simulink model "ACDCMG_woPV"  (R2020b)
settings: Solver=FixedStepAuto  StartTime=0.0  StopTime=0.2  FixedStep=Ts  MaxStep=1e-2  RelTol=1e-3
InitFcn:
  | Set_parameters_R2018
undefined symbols (not defined in the file): D1, D_invs, Delta, dis11, dis14, dis2, dis3, dis4, dis5, dis6, dis8, DiscIntNeverNeededParam, ee_sli_rtmsupport, fn, Fnom, gcbh, H_invs, Ion, Lithium, max_min, P_Load_3, P_nom_inv, Pnom_T1, Pnom_T2, Pnom_T3, Ql_Load_3, R_Load_9, R_Load_DC, Rl, Rls, S, sigbuilder_block, Ts, Ts_Control, Ts_Power, V1_LL_T3, VnInv, Vnom_DC, Vnom_Diesel, Vnom_prim, Vnom_sec, Vnom_ter_AC_DC, Xl, Xls
libraries: powerlib x238, powerlib_meascontrol x103, powerlib_extras x55, simulink x21, pid_lib x4, eeGeneralControl x2, re_lib x1, electricdrivelib x1, eeSinusoidalMeasurementV2 x1, eePowerMeasurement x1
(part 5 of 9)

== system ACDCMG_woPV/Grid Bi-directional Converter 1.2 300 (DC) // 150 V (AC) P_nom 3kW/Control of Inverter ==
  note: VL-L rms_2
  note: Primary control
  note: Control of Inverter
  Bus Selector : BusSelector  Commented=on  OutputSignals=signal1,signal2,signal3,signal4
  Demux3 : Demux  Outputs=3
  Demux4 : Demux  Outputs=3
  Discrete PWM Generator1 : Subsystem  Commented=on  AncestorBlock=|  DialogController=POWERSYS.PowerSysDialog  mask(Discrete PWM Generator){GeneratorMode=3-arm  bridge (6 pulses), Fc=4000, Ts=Ts_Power, Internal=off, mIndex=0.99, Freq=60, Phase=0}
      | powerlib_extras/Discrete 
      | Control Blocks/Discrete
      | PWM Generator
      mask prompts: GeneratorMode "Generator Mode"; Fc "Carrier frequency (Hz):"; Ts "Sample time:"; Internal "Internal generation of modulating signal(s)"; mIndex "Modulation index  (0<m<1) :"; Freq "Frequency of output voltage (Hz)"; Phase "Phase of output voltage (degrees)"
      mask help:
      | This discrete block generates pulses for carrier-based PWM (Pulse Width Modulation), self-commutated IGBTs,GTOs or FETs bridges.
      |
      | Depending on the number of bridge arms selected in the "Generator Mode" parameter, the block can be used either for single-phase or three-phase PWM control.
      mask init: same as ACDCMG_woPV/Grid Bi-directional Converter 1.1 300 (DC) // 150 V (AC) P_nom 3kW/Control of Inverter/Discrete PWM Generator1
      mask Help:
      | The output pulses are a vector (with values=0 or 1). Depending on the selected "Generator Mode", the output vector contains:
      | For a 1-arm  bridge: Two pulses. Pulse 1 is for the upper switch and pulse 2 is for the lower switch.
      | For a 2-arm  bridge: Four pulses. Pulses 1 and 3 are respectively for the upper switches of the first and second arm. Pulses 2 and 4 are for the lower switches.
      | For a 3-arm  bridge: Six pulses. Pulses 1,3 and 5 are respectively for the upper switches of the first,second and third arm. Pulses 2,4 and 6 are for the lower switches.
      | For double 3-arm bridges: Twelve pulses.The first six pulses (pulses 1 to 6) must be sent to the first 3-arm bridge and the last six (pulses 7 to 12) to the second 3-arm bridge.
      | 
      | By selecting "Internal generation" you can can control the modulation index m, frequency and phase of the output voltage  from the internal parameters (m, Freq and Phase). Otherwise, external signals are used for pulse generation. The width of the input vector must be 1 for single phase bridges ( 1-arm or 2-arm)  and 3 for 3-phase bridges  (single or double bridge).
      mask TypeOptions GeneratorMode: 1-arm  bridge (2 pulses) | 2-arm  bridge (4 pulses) | 3-arm  bridge (6 pulses) | Double 3-arm  bridges (12 pulses)
      mask Callback Internal: powericon('psbcallbacks',gcb,'Discrete PWM Generator',[]);
  Goto : Goto  Commented=on  GotoTag=PWM
  MI Controller : Subsystem  Commented=on
  Mux2 : Mux  Inputs=2
  PQ_B1 : Scope
  "P_Q(kW, kvar)1" : Display
      settings: Format=bank  Decimation=2000
  Positive-Sequence Active & Reactive Power1 : Subsystem  AncestorBlock=|  DialogController=POWERSYS.PowerSysDialog  mask(Discrete 3-phase Positive-Sequence Active & Reactive Power){Freq=60, Par_Vinit=[0 0], Par_Iinit=[0 0], Ts=5e-6}
      | powerlib_extras/Discrete
      | Measurements/Discrete 3-phase 
      | Positive-Sequence 
      | Active & Reactive Power
      mask prompts: Freq "Fundamental frequency (Hz):"; Par_Vinit "Voltage initial input: [ Mag  Phase(degrees) ]"; Par_Iinit "Current initial input: [ Mag  Phase(degrees) ]"; Ts "Sample time:"
      mask help:
      | Measure the three-phase active power P and reactive power Q associated with a periodic set of three-phase voltages and currents which may contain harmonics. P and Q are calculated by evaluating the fundamental values (positive-sequence) of the input voltages and currents with a running window over one cycle of the fundamental frequency.
      |
      | Current flowing into an RL circuit will produce  positive active and reactive powers.
      |
      | Vabc input: Three-phase instantaneous voltage (V)
      | Iabc input: Three-phase instantaneous current (A)
      |
      | Output 1: Vector [Mag_V(V) Mag_I(A)] of the fundamental values of the voltage & current (peak values of the positive-sequence)
      | Output 2: 3-phase PQ measurement vector [P(W) Q (var)] evaluated at the fundamental frequency.
      |
      | For the first cycle of simulation, the outputs are held constant using the values specified by the parameters "Initial input".
      mask init:
      | power_initmask();
      mask Help: This block is part of a subset of blocks in the Extras library that does not have documentation associated with it, other than the block mask description.
      mask Display: disp('')
  RMS_VI2 : Scope
  RMS_V_I1 : Display
      settings: Format=bank  Decimation=2000
  Scope1 : Scope  NumInputPorts=2
  Scope2 : Scope
  Scope6 : Scope  NumInputPorts=2
  Terminator{1..6} (6 alike) : Terminator
  Unit Delay4 : UnitDelay  Commented=on  SampleTime=Ts_Power  HasFrameUpgradeWarning=on
  V/F : Subsystem
  VL-L_2 : Scope  Commented=on  NumInputPorts=2
  Vph_rms_2 : Scope  Commented=on
  m2 : Scope  Commented=on
  m_2 : Scope  Commented=on
  Pulses : Outport  VectorParamsAs1DForOutWhenUnconnected=off
  wires:
  MI Controller/2(m) -> m_2/1
  Discrete PWM Generator1/1(Pulses) -> Unit Delay4/1
  MI Controller/1(Vabc_inv) -> Discrete PWM Generator1/1(Uref)
  Bus Selector/1 -> m2/1, MI Controller/1(Vabc)  "<signal1>"
  Bus Selector/2 -> VL-L_2/1  "<signal2>"
  Bus Selector/3 -> VL-L_2/2  "<signal3>"
  Bus Selector/4 -> Vph_rms_2/1  "<signal4>"
  [Udc] -> V/F/4(Udc)
  Demux3/2 -> Terminator1/1
  Demux4/3 -> Terminator6/1
  [i] -> V/F/3(i)
  Demux4/2 -> Terminator5/1
  Demux4/1 -> Mux2/2
  Demux3/3 -> Terminator4/1
  [io] -> Scope1/2, Positive-Sequence Active & Reactive Power1/2(Iabc)
  Mux2/1 -> Scope2/1
  Demux3/1 -> Mux2/1
  Positive-Sequence Active & Reactive Power1/2(P_Q(kW)) -> PQ_B1/1, "P_Q(kW, kvar)1"/1
  Positive-Sequence Active & Reactive Power1/4(PF) -> Terminator3/1
  Positive-Sequence Active & Reactive Power1/3(Phase_V_I) -> Terminator2/1
  Positive-Sequence Active & Reactive Power1/1(RMS_V_I) -> RMS_V_I1/1, RMS_VI2/1
  [e] -> Scope1/1, Positive-Sequence Active & Reactive Power1/1(Vabc)
  [e] -> Scope6/1, Demux3/1, V/F/1(e)
  [io] -> Scope6/2, Demux4/1, V/F/2(io)
  V/F/1(Pulses) -> Pulses/1

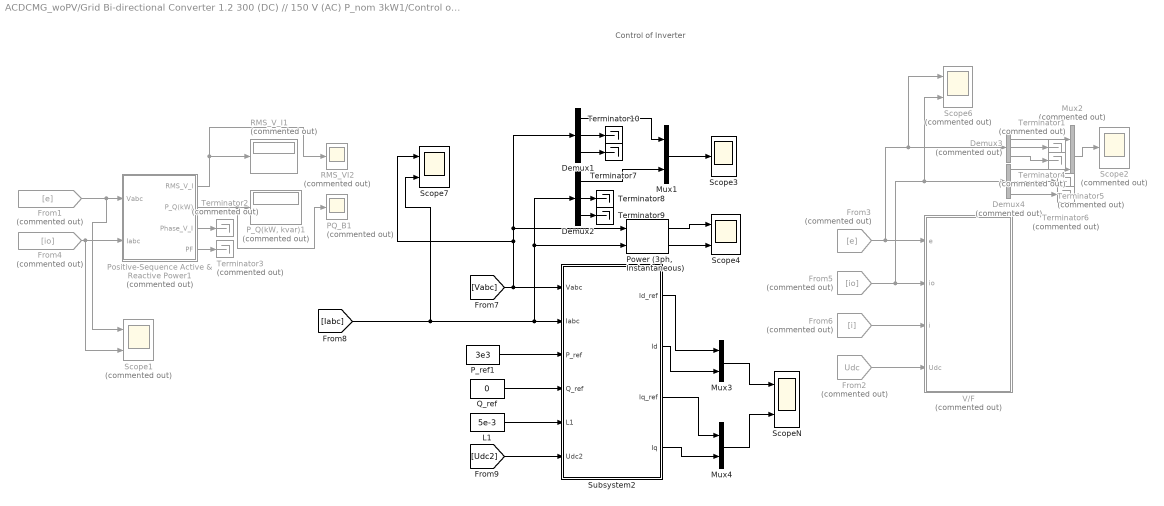
== system ACDCMG_woPV/Grid Bi-directional Converter 1.2 300 (DC) // 150 V (AC) P_nom 3kW1/Control of Inverter ==
  note: Control of Inverter
  Demux1 : Demux  Outputs=3
  Demux2 : Demux  Outputs=3
  Demux3 : Demux  Commented=on  Outputs=3
  Demux4 : Demux  Commented=on  Outputs=3
  From1 : From  Commented=on  GotoTag=e  TagVisibility=global
      settings: CloseFcn=tagdialog Close
  From2 : From  Commented=on  GotoTag=Udc  TagVisibility=global
  From3 : From  Commented=on  GotoTag=e  TagVisibility=global
  From4 : From  Commented=on  GotoTag=io  TagVisibility=global
      settings: CloseFcn=tagdialog Close
  From5 : From  Commented=on  GotoTag=io  TagVisibility=global
  From6 : From  Commented=on  GotoTag=i  TagVisibility=global
  L1 : Constant  Value=5e-3
  Mux1 : Mux  Inputs=2
  Mux2 : Mux  Commented=on  Inputs=2
  Mux3 : Mux  Inputs=2
  Mux4 : Mux  Inputs=2
  PQ_B1 : Scope  Commented=on
  "P_Q(kW, kvar)1" : Display  Commented=on
      settings: Format=bank  Decimation=2000
  P_ref1 : Constant  Value=3e3
  Positive-Sequence Active & Reactive Power1 : Subsystem  Commented=on  AncestorBlock=|  DialogController=POWERSYS.PowerSysDialog  mask(Discrete 3-phase Positive-Sequence Active & Reactive Power){Freq=60, Par_Vinit=[0 0], Par_Iinit=[0 0], Ts=5e-6}
      | powerlib_extras/Discrete
      | Measurements/Discrete 3-phase 
      | Positive-Sequence 
      | Active & Reactive Power
      mask prompts: Freq "Fundamental frequency (Hz):"; Par_Vinit "Voltage initial input: [ Mag  Phase(degrees) ]"; Par_Iinit "Current initial input: [ Mag  Phase(degrees) ]"; Ts "Sample time:"
      mask help:
      | Measure the three-phase active power P and reactive power Q associated with a periodic set of three-phase voltages and currents which may contain harmonics. P and Q are calculated by evaluating the fundamental values (positive-sequence) of the input voltages and currents with a running window over one cycle of the fundamental frequency.
      |
      | Current flowing into an RL circuit will produce  positive active and reactive powers.
      |
      | Vabc input: Three-phase instantaneous voltage (V)
      | Iabc input: Three-phase instantaneous current (A)
      |
      | Output 1: Vector [Mag_V(V) Mag_I(A)] of the fundamental values of the voltage & current (peak values of the positive-sequence)
      | Output 2: 3-phase PQ measurement vector [P(W) Q (var)] evaluated at the fundamental frequency.
      |
      | For the first cycle of simulation, the outputs are held constant using the values specified by the parameters "Initial input".
      mask init:
      | power_initmask();
      mask Help: This block is part of a subset of blocks in the Extras library that does not have documentation associated with it, other than the block mask description.
      mask Display: disp('')
  "Power (3ph, Instantaneous)" : powerlib_meascontrol/Measurements/Power (3ph, Instantaneous)
  Q_ref : Constant  Value=0
  RMS_VI2 : Scope  Commented=on
  RMS_V_I1 : Display  Commented=on
      settings: Format=bank  Decimation=2000
  Scope1 : Scope  Commented=on  NumInputPorts=2
  Scope2 : Scope  Commented=on
  Scope3 : Scope
  Scope4 : Scope  NumInputPorts=2
  Scope6 : Scope  Commented=on  NumInputPorts=2
  Scope7 : Scope  NumInputPorts=2
  ScopeN : Scope  NumInputPorts=2
  Subsystem2 : Subsystem  mask{Kp=21, Ki=101, Kd=0}
      mask prompts: Kp "Proportional gain (Kp):"; Ki "Integral gain (Ki):"; Kd "Derivative gain (Kd):"
  Terminator{1..6} (6 alike) : Terminator  Commented=on
  Terminator{7..10} (4 alike) : Terminator
  V/F : Subsystem  Commented=on
  wires:
  From2/1 -> V/F/4(Udc)
  Demux3/2 -> Terminator1/1
  Demux4/3 -> Terminator6/1
  From6/1 -> V/F/3(i)
  Demux4/2 -> Terminator5/1
  Demux4/1 -> Mux2/2
  Demux3/3 -> Terminator4/1
  From4/1 -> Scope1/2, Positive-Sequence Active & Reactive Power1/2(Iabc)
  Mux2/1 -> Scope2/1
  Demux3/1 -> Mux2/1
  Positive-Sequence Active & Reactive Power1/2(P_Q(kW)) -> PQ_B1/1, "P_Q(kW, kvar)1"/1
  Positive-Sequence Active & Reactive Power1/4(PF) -> Terminator3/1
  Positive-Sequence Active & Reactive Power1/3(Phase_V_I) -> Terminator2/1
  Positive-Sequence Active & Reactive Power1/1(RMS_V_I) -> RMS_V_I1/1, RMS_VI2/1
  From1/1 -> Scope1/1, Positive-Sequence Active & Reactive Power1/1(Vabc)
  From3/1 -> Scope6/1, Demux3/1, V/F/1(e)
  From5/1 -> Scope6/2, Demux4/1, V/F/2(io)
  Q_ref/1 -> Subsystem2/4(Q_ref)
  [Vabc] -> Subsystem2/1(Vabc), Scope7/1, Demux1/1, "Power (3ph, Instantaneous)"/1
  Demux2/3 -> Terminator9/1
  Demux1/2 -> Terminator10/1
  [Udc2] -> Subsystem2/6(Udc2)
  P_ref1/1 -> Subsystem2/3(P_ref)
  Demux2/2 -> Terminator8/1
  "Power (3ph, Instantaneous)"/2 -> Scope4/2
  "Power (3ph, Instantaneous)"/1 -> Scope4/1
  Subsystem2/3(Iq_ref) -> Mux4/1
  Subsystem2/2(Id) -> Mux3/2
  Demux2/1 -> Mux1/2
  Mux1/1 -> Scope3/1
  L1/1 -> Subsystem2/5(L1)
  Mux3/1 -> ScopeN/1
  Subsystem2/4(Iq) -> Mux4/2
  [Iabc] -> Scope7/2, Demux2/1, "Power (3ph, Instantaneous)"/2, Subsystem2/2(Iabc)
  Subsystem2/1(Id_ref) -> Mux3/1
  Mux4/1 -> ScopeN/2
  Demux1/3 -> Terminator7/1
  Demux1/1 -> Mux1/1

== system ACDCMG_woPV/Grid Bi-directional Converter 1.2 300 (DC) // 150 V (AC) P_nom 3kW1/Power Measurement (Three-Phase) ==
  V : Inport
  I : Inport  Port=2
  Continuous : Subsystem  VariantControl=Continuous
  Discrete : Subsystem  VariantControl=Discrete
  P : Outport  VectorParamsAs1DForOutWhenUnconnected=off
  Q : Outport  Port=2  VectorParamsAs1DForOutWhenUnconnected=off

== system ACDCMG_woPV/Grid Bi-directional Converter 1.2 300 (DC) // 150 V (AC) P_nom 3kW2/Control of Inverter ==
  note: VL-L rms_2
  note: Primary control
  note: Control of Inverter
  Bus Selector : BusSelector  Commented=on  OutputSignals=signal1,signal2,signal3,signal4
  Demux3 : Demux  Outputs=3
  Demux4 : Demux  Outputs=3
  Discrete PWM Generator1 : Subsystem  Commented=on  AncestorBlock=|  DialogController=POWERSYS.PowerSysDialog  mask(Discrete PWM Generator){GeneratorMode=3-arm  bridge (6 pulses), Fc=4000, Ts=Ts_Power, Internal=off, mIndex=0.99, Freq=60, Phase=0}
      | powerlib_extras/Discrete 
      | Control Blocks/Discrete
      | PWM Generator
      mask prompts: GeneratorMode "Generator Mode"; Fc "Carrier frequency (Hz):"; Ts "Sample time:"; Internal "Internal generation of modulating signal(s)"; mIndex "Modulation index  (0<m<1) :"; Freq "Frequency of output voltage (Hz)"; Phase "Phase of output voltage (degrees)"
      mask help:
      | This discrete block generates pulses for carrier-based PWM (Pulse Width Modulation), self-commutated IGBTs,GTOs or FETs bridges.
      |
      | Depending on the number of bridge arms selected in the "Generator Mode" parameter, the block can be used either for single-phase or three-phase PWM control.
      mask init: same as ACDCMG_woPV/Grid Bi-directional Converter 1.1 300 (DC) // 150 V (AC) P_nom 3kW/Control of Inverter/Discrete PWM Generator1
      mask Help:
      | The output pulses are a vector (with values=0 or 1). Depending on the selected "Generator Mode", the output vector contains:
      | For a 1-arm  bridge: Two pulses. Pulse 1 is for the upper switch and pulse 2 is for the lower switch.
      | For a 2-arm  bridge: Four pulses. Pulses 1 and 3 are respectively for the upper switches of the first and second arm. Pulses 2 and 4 are for the lower switches.
      | For a 3-arm  bridge: Six pulses. Pulses 1,3 and 5 are respectively for the upper switches of the first,second and third arm. Pulses 2,4 and 6 are for the lower switches.
      | For double 3-arm bridges: Twelve pulses.The first six pulses (pulses 1 to 6) must be sent to the first 3-arm bridge and the last six (pulses 7 to 12) to the second 3-arm bridge.
      | 
      | By selecting "Internal generation" you can can control the modulation index m, frequency and phase of the output voltage  from the internal parameters (m, Freq and Phase). Otherwise, external signals are used for pulse generation. The width of the input vector must be 1 for single phase bridges ( 1-arm or 2-arm)  and 3 for 3-phase bridges  (single or double bridge).
      mask TypeOptions GeneratorMode: 1-arm  bridge (2 pulses) | 2-arm  bridge (4 pulses) | 3-arm  bridge (6 pulses) | Double 3-arm  bridges (12 pulses)
      mask Callback Internal: powericon('psbcallbacks',gcb,'Discrete PWM Generator',[]);
  Goto : Goto  Commented=on  GotoTag=PWM
  MI Controller : Subsystem  Commented=on
  Mux2 : Mux  Inputs=2
  PQ_B1 : Scope
  "P_Q(kW, kvar)1" : Display
      settings: Format=bank  Decimation=2000
  Positive-Sequence Active & Reactive Power1 : Subsystem  AncestorBlock=|  DialogController=POWERSYS.PowerSysDialog  mask(Discrete 3-phase Positive-Sequence Active & Reactive Power){Freq=60, Par_Vinit=[0 0], Par_Iinit=[0 0], Ts=5e-6}
      | powerlib_extras/Discrete
      | Measurements/Discrete 3-phase 
      | Positive-Sequence 
      | Active & Reactive Power
      mask prompts: Freq "Fundamental frequency (Hz):"; Par_Vinit "Voltage initial input: [ Mag  Phase(degrees) ]"; Par_Iinit "Current initial input: [ Mag  Phase(degrees) ]"; Ts "Sample time:"
      mask help:
      | Measure the three-phase active power P and reactive power Q associated with a periodic set of three-phase voltages and currents which may contain harmonics. P and Q are calculated by evaluating the fundamental values (positive-sequence) of the input voltages and currents with a running window over one cycle of the fundamental frequency.
      |
      | Current flowing into an RL circuit will produce  positive active and reactive powers.
      |
      | Vabc input: Three-phase instantaneous voltage (V)
      | Iabc input: Three-phase instantaneous current (A)
      |
      | Output 1: Vector [Mag_V(V) Mag_I(A)] of the fundamental values of the voltage & current (peak values of the positive-sequence)
      | Output 2: 3-phase PQ measurement vector [P(W) Q (var)] evaluated at the fundamental frequency.
      |
      | For the first cycle of simulation, the outputs are held constant using the values specified by the parameters "Initial input".
      mask init:
      | power_initmask();
      mask Help: This block is part of a subset of blocks in the Extras library that does not have documentation associated with it, other than the block mask description.
      mask Display: disp('')
  RMS_VI2 : Scope
  RMS_V_I1 : Display
      settings: Format=bank  Decimation=2000
  Scope1 : Scope  NumInputPorts=2
  Scope2 : Scope
  Scope6 : Scope  NumInputPorts=2
  Terminator{1..6} (6 alike) : Terminator
  Unit Delay4 : UnitDelay  Commented=on  SampleTime=Ts_Power  HasFrameUpgradeWarning=on
  V/F : Subsystem
  VL-L_2 : Scope  Commented=on  NumInputPorts=2
  Vph_rms_2 : Scope  Commented=on
  m2 : Scope  Commented=on
  m_2 : Scope  Commented=on
  Pulses : Outport  VectorParamsAs1DForOutWhenUnconnected=off
  wires:
  MI Controller/2(m) -> m_2/1
  Discrete PWM Generator1/1(Pulses) -> Unit Delay4/1
  MI Controller/1(Vabc_inv) -> Discrete PWM Generator1/1(Uref)
  Bus Selector/1 -> m2/1, MI Controller/1(Vabc)  "<signal1>"
  Bus Selector/2 -> VL-L_2/1  "<signal2>"
  Bus Selector/3 -> VL-L_2/2  "<signal3>"
  Bus Selector/4 -> Vph_rms_2/1  "<signal4>"
  [Udc] -> V/F/4(Udc)
  Demux3/2 -> Terminator1/1
  Demux4/3 -> Terminator6/1
  [i] -> V/F/3(i)
  Demux4/2 -> Terminator5/1
  Demux4/1 -> Mux2/2
  Demux3/3 -> Terminator4/1
  [io] -> Scope1/2, Positive-Sequence Active & Reactive Power1/2(Iabc)
  Mux2/1 -> Scope2/1
  Demux3/1 -> Mux2/1
  Positive-Sequence Active & Reactive Power1/2(P_Q(kW)) -> PQ_B1/1, "P_Q(kW, kvar)1"/1
  Positive-Sequence Active & Reactive Power1/4(PF) -> Terminator3/1
  Positive-Sequence Active & Reactive Power1/3(Phase_V_I) -> Terminator2/1
  Positive-Sequence Active & Reactive Power1/1(RMS_V_I) -> RMS_V_I1/1, RMS_VI2/1
  [e] -> Scope1/1, Positive-Sequence Active & Reactive Power1/1(Vabc)
  [e] -> Scope6/1, Demux3/1, V/F/1(e)
  [io] -> Scope6/2, Demux4/1, V/F/2(io)
  V/F/1(Pulses) -> Pulses/1

== system ACDCMG_woPV/Grid Bi-directional Converter 1.2 300 (DC) // 150 V (AC) P_nom 3kW3/Control of Inverter ==
  note: Control of Inverter
  Demux3 : Demux  Outputs=3
  Demux4 : Demux  Outputs=3
  From1 : From  Commented=on  GotoTag=e  TagVisibility=global
      settings: CloseFcn=tagdialog Close
  From4 : From  Commented=on  GotoTag=io  TagVisibility=global
      settings: CloseFcn=tagdialog Close
  Mux2 : Mux  Inputs=2
  PQ_B1 : Scope  Commented=on
  "P_Q(kW, kvar)1" : Display  Commented=on
      settings: Format=bank  Decimation=2000
  Positive-Sequence Active & Reactive Power1 : Subsystem  Commented=on  AncestorBlock=|  DialogController=POWERSYS.PowerSysDialog  mask(Discrete 3-phase Positive-Sequence Active & Reactive Power){Freq=60, Par_Vinit=[0 0], Par_Iinit=[0 0], Ts=5e-6}
      | powerlib_extras/Discrete
      | Measurements/Discrete 3-phase 
      | Positive-Sequence 
      | Active & Reactive Power
      mask prompts: Freq "Fundamental frequency (Hz):"; Par_Vinit "Voltage initial input: [ Mag  Phase(degrees) ]"; Par_Iinit "Current initial input: [ Mag  Phase(degrees) ]"; Ts "Sample time:"
      mask help:
      | Measure the three-phase active power P and reactive power Q associated with a periodic set of three-phase voltages and currents which may contain harmonics. P and Q are calculated by evaluating the fundamental values (positive-sequence) of the input voltages and currents with a running window over one cycle of the fundamental frequency.
      |
      | Current flowing into an RL circuit will produce  positive active and reactive powers.
      |
      | Vabc input: Three-phase instantaneous voltage (V)
      | Iabc input: Three-phase instantaneous current (A)
      |
      | Output 1: Vector [Mag_V(V) Mag_I(A)] of the fundamental values of the voltage & current (peak values of the positive-sequence)
      | Output 2: 3-phase PQ measurement vector [P(W) Q (var)] evaluated at the fundamental frequency.
      |
      | For the first cycle of simulation, the outputs are held constant using the values specified by the parameters "Initial input".
      mask init:
      | power_initmask();
      mask Help: This block is part of a subset of blocks in the Extras library that does not have documentation associated with it, other than the block mask description.
      mask Display: disp('')
  RMS_VI2 : Scope  Commented=on
  RMS_V_I1 : Display  Commented=on
      settings: Format=bank  Decimation=2000
  Scope1 : Scope  Commented=on  NumInputPorts=2
  Scope2 : Scope
  Scope6 : Scope  NumInputPorts=2
  Terminator{1,4..6} (4 alike) : Terminator
  Terminator2 : Terminator  Commented=on
  Terminator3 : Terminator  Commented=on
  V/F : Subsystem
  wires:
  [Udc] -> V/F/4(Udc)
  Demux3/2 -> Terminator1/1
  Demux4/3 -> Terminator6/1
  [i] -> V/F/3(i)
  Demux4/2 -> Terminator5/1
  Demux4/1 -> Mux2/2
  Demux3/3 -> Terminator4/1
  From4/1 -> Scope1/2, Positive-Sequence Active & Reactive Power1/2(Iabc)
  Mux2/1 -> Scope2/1
  Demux3/1 -> Mux2/1
  Positive-Sequence Active & Reactive Power1/2(P_Q(kW)) -> PQ_B1/1, "P_Q(kW, kvar)1"/1
  Positive-Sequence Active & Reactive Power1/4(PF) -> Terminator3/1
  Positive-Sequence Active & Reactive Power1/3(Phase_V_I) -> Terminator2/1
  Positive-Sequence Active & Reactive Power1/1(RMS_V_I) -> RMS_V_I1/1, RMS_VI2/1
  From1/1 -> Scope1/1, Positive-Sequence Active & Reactive Power1/1(Vabc)
  [e] -> Scope6/1, Demux3/1, V/F/1(e)
  [io] -> Scope6/2, Demux4/1, V/F/2(io)

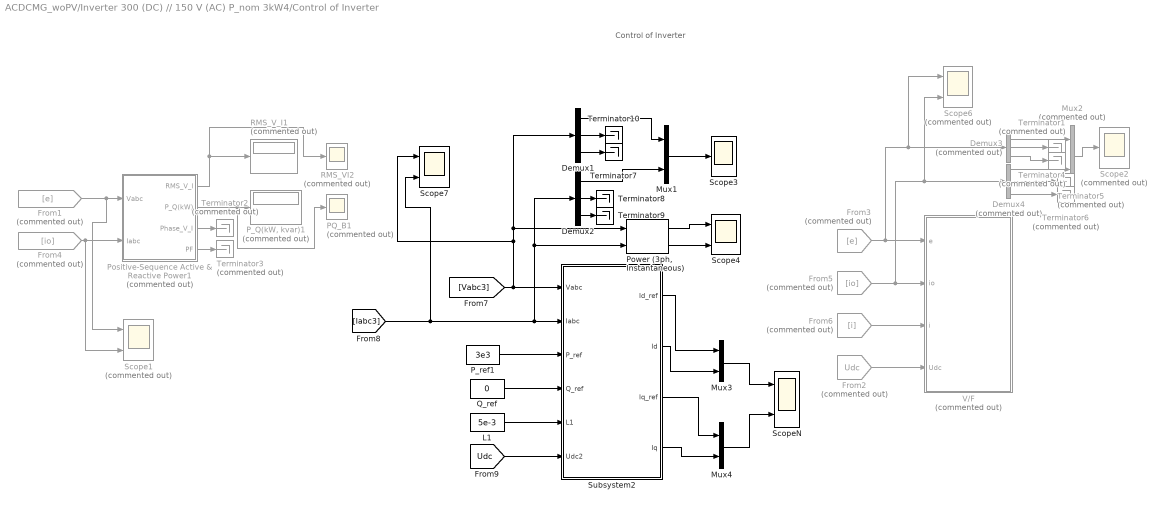
== system ACDCMG_woPV/Inverter 300 (DC) // 150 V (AC) P_nom 3kW4/Control of Inverter ==
  note: Control of Inverter
  Demux1 : Demux  Outputs=3
  Demux2 : Demux  Outputs=3
  Demux3 : Demux  Commented=on  Outputs=3
  Demux4 : Demux  Commented=on  Outputs=3
  From1 : From  Commented=on  GotoTag=e  TagVisibility=global
      settings: CloseFcn=tagdialog Close
  From2 : From  Commented=on  GotoTag=Udc  TagVisibility=global
  From3 : From  Commented=on  GotoTag=e  TagVisibility=global
  From4 : From  Commented=on  GotoTag=io  TagVisibility=global
      settings: CloseFcn=tagdialog Close
  From5 : From  Commented=on  GotoTag=io  TagVisibility=global
  From6 : From  Commented=on  GotoTag=i  TagVisibility=global
  L1 : Constant  Value=5e-3
  Mux1 : Mux  Inputs=2
  Mux2 : Mux  Commented=on  Inputs=2
  Mux3 : Mux  Inputs=2
  Mux4 : Mux  Inputs=2
  PQ_B1 : Scope  Commented=on
  "P_Q(kW, kvar)1" : Display  Commented=on
      settings: Format=bank  Decimation=2000
  P_ref1 : Constant  Value=3e3
  Positive-Sequence Active & Reactive Power1 : Subsystem  Commented=on  AncestorBlock=|  DialogController=POWERSYS.PowerSysDialog  mask(Discrete 3-phase Positive-Sequence Active & Reactive Power){Freq=60, Par_Vinit=[0 0], Par_Iinit=[0 0], Ts=5e-6}
      | powerlib_extras/Discrete
      | Measurements/Discrete 3-phase 
      | Positive-Sequence 
      | Active & Reactive Power
      mask prompts: Freq "Fundamental frequency (Hz):"; Par_Vinit "Voltage initial input: [ Mag  Phase(degrees) ]"; Par_Iinit "Current initial input: [ Mag  Phase(degrees) ]"; Ts "Sample time:"
      mask help:
      | Measure the three-phase active power P and reactive power Q associated with a periodic set of three-phase voltages and currents which may contain harmonics. P and Q are calculated by evaluating the fundamental values (positive-sequence) of the input voltages and currents with a running window over one cycle of the fundamental frequency.
      |
      | Current flowing into an RL circuit will produce  positive active and reactive powers.
      |
      | Vabc input: Three-phase instantaneous voltage (V)
      | Iabc input: Three-phase instantaneous current (A)
      |
      | Output 1: Vector [Mag_V(V) Mag_I(A)] of the fundamental values of the voltage & current (peak values of the positive-sequence)
      | Output 2: 3-phase PQ measurement vector [P(W) Q (var)] evaluated at the fundamental frequency.
      |
      | For the first cycle of simulation, the outputs are held constant using the values specified by the parameters "Initial input".
      mask init:
      | power_initmask();
      mask Help: This block is part of a subset of blocks in the Extras library that does not have documentation associated with it, other than the block mask description.
      mask Display: disp('')
  "Power (3ph, Instantaneous)" : powerlib_meascontrol/Measurements/Power (3ph, Instantaneous)
  Q_ref : Constant  Value=0
  RMS_VI2 : Scope  Commented=on
  RMS_V_I1 : Display  Commented=on
      settings: Format=bank  Decimation=2000
  Scope1 : Scope  Commented=on  NumInputPorts=2
  Scope2 : Scope  Commented=on
  Scope3 : Scope
  Scope4 : Scope  NumInputPorts=2
  Scope6 : Scope  Commented=on  NumInputPorts=2
  Scope7 : Scope  NumInputPorts=2
  ScopeN : Scope  NumInputPorts=2
  Subsystem2 : Subsystem  mask{Kp=21, Ki=101, Kd=0}
      mask prompts: Kp "Proportional gain (Kp):"; Ki "Integral gain (Ki):"; Kd "Derivative gain (Kd):"
  Terminator{1..6} (6 alike) : Terminator  Commented=on
  Terminator{7..10} (4 alike) : Terminator
  V/F : Subsystem  Commented=on
  wires:
  From2/1 -> V/F/4(Udc)
  Demux3/2 -> Terminator1/1
  Demux4/3 -> Terminator6/1
  From6/1 -> V/F/3(i)
  Demux4/2 -> Terminator5/1
  Demux4/1 -> Mux2/2
  Demux3/3 -> Terminator4/1
  From4/1 -> Scope1/2, Positive-Sequence Active & Reactive Power1/2(Iabc)
  Mux2/1 -> Scope2/1
  Demux3/1 -> Mux2/1
  Positive-Sequence Active & Reactive Power1/2(P_Q(kW)) -> PQ_B1/1, "P_Q(kW, kvar)1"/1
  Positive-Sequence Active & Reactive Power1/4(PF) -> Terminator3/1
  Positive-Sequence Active & Reactive Power1/3(Phase_V_I) -> Terminator2/1
  Positive-Sequence Active & Reactive Power1/1(RMS_V_I) -> RMS_V_I1/1, RMS_VI2/1
  From1/1 -> Scope1/1, Positive-Sequence Active & Reactive Power1/1(Vabc)
  From3/1 -> Scope6/1, Demux3/1, V/F/1(e)
  From5/1 -> Scope6/2, Demux4/1, V/F/2(io)
  Q_ref/1 -> Subsystem2/4(Q_ref)
  [Vabc3] -> Subsystem2/1(Vabc), Scope7/1, Demux1/1, "Power (3ph, Instantaneous)"/1
  Demux2/3 -> Terminator9/1
  Demux1/2 -> Terminator10/1
  [Udc] -> Subsystem2/6(Udc2)
  P_ref1/1 -> Subsystem2/3(P_ref)
  Demux2/2 -> Terminator8/1
  "Power (3ph, Instantaneous)"/2 -> Scope4/2
  "Power (3ph, Instantaneous)"/1 -> Scope4/1
  Subsystem2/3(Iq_ref) -> Mux4/1
  Subsystem2/2(Id) -> Mux3/2
  Demux2/1 -> Mux1/2
  Mux1/1 -> Scope3/1
  L1/1 -> Subsystem2/5(L1)
  Mux3/1 -> ScopeN/1
  Subsystem2/4(Iq) -> Mux4/2
  [Iabc3] -> Scope7/2, Demux2/1, "Power (3ph, Instantaneous)"/2, Subsystem2/2(Iabc)
  Subsystem2/1(Id_ref) -> Mux3/1
  Mux4/1 -> ScopeN/2
  Demux1/3 -> Terminator7/1
  Demux1/1 -> Mux1/1

== system ACDCMG_woPV/Load_2/Power Factor Block1 ==
  Vabc : Inport
  Iabc : Inport  Port=2
  Complex to Magnitude-Angle : ComplexToMagnitudeAngle  Commented=on
  Power : powerlib_meascontrol/Measurements/Power  Commented=on  Freq=Freq  Vinit=Vinit  Iinit=Iinit  Ts=Ts
  Real-Imag to Complex : RealImagToComplex  Commented=on
  Terminator : Terminator  Commented=on
  cos(theta) : Trigonometry  Commented=on  Operator=cos
  Vabc y Vabc : Outport  VectorParamsAs1DForOutWhenUnconnected=off
  "Iabc y Iabc " : Outport  Port=2  VectorParamsAs1DForOutWhenUnconnected=off
  wires:
  Power/1 -> Real-Imag to Complex/1
  Power/2 -> Real-Imag to Complex/2
  Complex to Magnitude-Angle/2 -> cos(theta)/1
  Real-Imag to Complex/1 -> Complex to Magnitude-Angle/1
  cos(theta)/1 -> ?
  Complex to Magnitude-Angle/1 -> Terminator/1
  Iabc/1 -> "Iabc y Iabc "/1, Power/2
  Vabc/1 -> Vabc y Vabc/1, Power/1

== system ACDCMG_woPV/Resource1/Irradiance Temp Demand Max ==
  Demux : Demux  Tag=STV Demux  Outputs=2
      settings: DisplayOption=none
  FromWs : FromWorkspace  Tag=STV FromWs  VariableName=tuvar
      SigBuilderData=|
      | common.afterFinalStr = 'Extrapolate'
      | common.sampleTime = '0'
      | dataSet(1).timeRange = [0 2]
      | dataSet(1).name = 'Constant Irradiance'
      | dataSet(2).timeRange = [0 2]
      | dataSet(2).name = 'Step Irradiance'
      | dataSet(3).timeRange = [0 3]
      | dataSet(3).name = 'Ramp-up/down Irradiance'
      | sbobj.Groups(1).Name = 'Constant Irradiance'
      | sbobj.Groups(1).Signals(1).Name = 'Ir'
      | sbobj.Groups(1).Signals(1).XData = [0 2]
      | sbobj.Groups(1).Signals(1).YData = [1000 1000]
      | sbobj.Groups(1).Signals(2).Name = 'Temp'
      | sbobj.Groups(1).Signals(2).XData = [0 1 1 2]
      | sbobj.Groups(1).Signals(2).YData = [0 0 1 1]
      | sbobj.Groups(1).TimeRange = [0 2]
      | sbobj.Groups(2).Name = 'Step Irradiance'
      | sbobj.Groups(2).Signals(1).Name = 'Ir'
      | sbobj.Groups(2).Signals(1).XData = [0 0.252 0.252 2]
      | sbobj.Groups(2).Signals(1).YData = [600 600 1000 1000]
      | sbobj.Groups(2).Signals(2).Name = 'Temp'
      | sbobj.Groups(2).Signals(2).XData = [0 1 1 2]
      | sbobj.Groups(2).Signals(2).YData = [0 0 1 1]
      | sbobj.Groups(2).TimeRange = [0 2]
      | sbobj.Groups(3).Name = 'Ramp-up/down Irradiance'
      | sbobj.Groups(3).Signals(1).Name = 'Ir'
      | sbobj.Groups(3).Signals(1).XData = [0 0.785 1.7 2.28 3]
      | sbobj.Groups(3).Signals(1).YData = [1000 999.538235294 999 999.446153846 1000]
      | sbobj.Groups(3).Signals(2).Name = 'Temp'
      | sbobj.Groups(3).Signals(2).XData = [0 2 2.1 3]
      | sbobj.Groups(3).Signals(2).YData = [25 25 25 25]
      | sbobj.Groups(3).TimeRange = [0 3]
  Ir : Outport  Tag=STV Outport  VectorParamsAs1DForOutWhenUnconnected=off
  Temp : Outport  Tag=STV Outport  Port=2  VectorParamsAs1DForOutWhenUnconnected=off
  wires:
  Demux/1 -> Ir/1
  FromWs/1 -> Demux/1
  Demux/2 -> Temp/1

== system ACDCMG_woPV/Boost -buck Bi-directional converter 1 0.65 kW/+ve reference For Buck --> -ve reference For Boost <--/PID Orig Boost ==
  error : Inport
  Integrator2 : Integrator  LimitOutput=on  UpperSaturationLimit=0.9  LowerSaturationLimit=0
  Ki2 : Gain  Gain=3
  Kp2 : Gain  Gain=0.02
  Sum4 : Sum  Inputs=|++
  Out1 : Outport  VectorParamsAs1DForOutWhenUnconnected=off
  wires:
  error/1 -> Kp2/1, Ki2/1
  Kp2/1 -> Sum4/1
  Sum4/1 -> Out1/1
  Ki2/1 -> Integrator2/1
  Integrator2/1 -> Sum4/2

== system ACDCMG_woPV/Boost -buck Bi-directional converter 1 0.65 kW/+ve reference For Buck --> -ve reference For Boost <--/PID Orig Buck ==
  error : Inport
  Integrator3 : Integrator  LimitOutput=on  UpperSaturationLimit=0.9  LowerSaturationLimit=0
  Ki3 : Gain  Gain=110
  Kp3 : Gain  Gain=0.2
  Sum1 : Sum  Inputs=|++
  Out1 : Outport  VectorParamsAs1DForOutWhenUnconnected=off
  wires:
  Integrator3/1 -> Sum1/2
  Ki3/1 -> Integrator3/1
  Kp3/1 -> Sum1/1
  Sum1/1 -> Out1/1
  error/1 -> Kp3/1, Ki3/1

== system ACDCMG_woPV/Boost -buck Bi-directional converter 1 0.65 kW/Primary Control/PID Orig Boost ==
  error : Inport
  Delay : Delay  DelayLength=1  InitialCondition=0  SampleTime=Ts
  Integrator : Integrator  InitialCondition=0.1  LimitOutput=on  UpperSaturationLimit=0.9  LowerSaturationLimit=0.1
  Ki : Gain  Gain=0.001
  Kp : Gain  Gain=0.000005
  Kp1 : Gain  Gain=60
  Sum1 : Sum  Inputs=|++
  Out1 : Outport  VectorParamsAs1DForOutWhenUnconnected=off
  wires:
  Integrator/1 -> Sum1/2
  Sum1/1 -> Out1/1
  Ki/1 -> Integrator/1
  Kp/1 -> Sum1/1
  error/1 -> Delay/1
  Delay/1 -> Kp1/1
  Kp1/1 -> Kp/1, Ki/1

== system ACDCMG_woPV/Boost -buck Bi-directional converter DC //DC 1 0.65 kW Switching Model/+ve reference For Buck --> -ve reference For Boost <--/PID Orig Boost ==
  error : Inport
  Integrator2 : Integrator  LimitOutput=on  UpperSaturationLimit=0.9  LowerSaturationLimit=0
  Ki2 : Gain  Gain=3
  Kp2 : Gain  Gain=0.02
  Sum4 : Sum  Inputs=|++
  Out1 : Outport  VectorParamsAs1DForOutWhenUnconnected=off
  wires:
  error/1 -> Kp2/1, Ki2/1
  Kp2/1 -> Sum4/1
  Sum4/1 -> Out1/1
  Ki2/1 -> Integrator2/1
  Integrator2/1 -> Sum4/2

== system ACDCMG_woPV/Boost -buck Bi-directional converter DC //DC 1 0.65 kW Switching Model/+ve reference For Buck --> -ve reference For Boost <--/PID Orig Buck ==
  error : Inport
  Integrator3 : Integrator  LimitOutput=on  UpperSaturationLimit=0.9  LowerSaturationLimit=0
  Ki3 : Gain  Gain=110
  Kp3 : Gain  Gain=0.2
  Sum1 : Sum  Inputs=|++
  Out1 : Outport  VectorParamsAs1DForOutWhenUnconnected=off
  wires:
  Integrator3/1 -> Sum1/2
  Ki3/1 -> Integrator3/1
  Kp3/1 -> Sum1/1
  Sum1/1 -> Out1/1
  error/1 -> Kp3/1, Ki3/1

== system ACDCMG_woPV/Boost -buck Bi-directional converter DC //DC 1 0.65 kW Switching Model/Primary Control/PID Orig Boost ==
  error : Inport
  Integrator : Integrator  LimitOutput=on  UpperSaturationLimit=0.9  LowerSaturationLimit=0
  Ki : Gain  Gain=3
  Kp : Gain  Gain=0.02
  Sum1 : Sum  Inputs=|++
  Out1 : Outport  VectorParamsAs1DForOutWhenUnconnected=off
  wires:
  Integrator/1 -> Sum1/2
  Sum1/1 -> Out1/1
  Ki/1 -> Integrator/1
  Kp/1 -> Sum1/1
  error/1 -> Ki/1, Kp/1

== system ACDCMG_woPV/Boost -buck Bi-directional converter DC //DC 1 0.65 kW Switching Model/Primary Control/PID Orig Buck ==
  error : Inport
  Integrator : Integrator  LimitOutput=on  UpperSaturationLimit=0.9  LowerSaturationLimit=0
  Ki : Gain  Gain=110
  Kp : Gain  Gain=0.02
  Sum1 : Sum  Inputs=|++
  Out1 : Outport  VectorParamsAs1DForOutWhenUnconnected=off
  wires:
  error/1 -> Kp/1, Ki/1
  Kp/1 -> Sum1/1
  Ki/1 -> Integrator/1
  Sum1/1 -> Out1/1
  Integrator/1 -> Sum1/2

== system ACDCMG_woPV/Boost converter DC //CD 2 5 kHz - 300V /MPPT Controller using  "Incremental Conductance + Integral Regulator "  technique /MPPT ==
  note: Maximum power point tracking by incremental conductance method
      | --------------------------------------------------------------
      | Maximum power point is obtained when dP/dV=0  where P= V*I
      | -> d(V*I)/dV = I + V*dI/dV = 0
      | -> dI/dV = -I/V
      |
      | dI, dV  = fundamental components of I and V ripples measured with a sliding time window T_MPPT
      | I , V   = mean values of V and I measured with a sliding time window T_MPPT
      |
      | The integral regulator minimizes the error (dI/dV + I/V)
      | Regulator output = Duty cycle correction
  V_PV : Inport
  I_PV : Inport  Port=2
  on/off : Inport  Port=3
  Add : Sum  Inputs=+-
  Add1 : Sum
  Constant : Constant  Value=0
  Constant1 : Constant  Value=0
  Dead Zone : DeadZone  LowerValue=-0.05  UpperValue=0.05  SaturateOnIntegerOverflow=on
  Discrete-Time Integrator : DiscreteIntegrator  SampleTime=Ts_Control  LimitOutput=on  UpperSaturationLimit=1  LowerSaturationLimit=-1  ICPrevOutput=DiscIntNeverNeededParam  ICPrevScaledInput=DiscIntNeverNeededParam
  Fourier : powerlib_meascontrol/Measurements/Fourier  Freq=1/T_MPPT  n=1  InInit=[0, 0]  Ts=Ts_Control
  Fourier1 : powerlib_meascontrol/Measurements/Fourier  Freq=1/T_MPPT  n=1  InInit=[0, 0]  Ts=Ts_Control
  Gain : Gain  Gain=-1
  MPPT Gain : Gain  Gain=5
  MPPT Algorithm : Scope
  Mean : powerlib_meascontrol/Measurements/Mean  Freq=1/T_MPPT  Vinit=0  Ts=Ts_Control
  Mean1 : powerlib_meascontrol/Measurements/Mean  Freq=1/T_MPPT  Vinit=0  Ts=Ts_Control
  Mux2 : Mux  Inputs=2
  Saturation : Saturate  UpperLimit=inf  LowerLimit=eps
  Saturation1 : Saturate  UpperLimit=inf  LowerLimit=eps
  Switch : Switch  Threshold=0.5
  Switch1 : Switch  Threshold=0.5
  Trigonometric Function : Trigonometry  Operator=cos
  deg2rad : Gain  Gain=pi/180
  div : Product  Inputs=*/  RndMeth=Zero
  div1 : Product  Inputs=**  RndMeth=Zero
  div2 : Product  Inputs=*/  RndMeth=Zero
  Delta_D : Outport  VectorParamsAs1DForOutWhenUnconnected=off
  tag scope: I_V_MPPT=global, Imean_PV=global, Vmean_PV=global, dI_dV_MPPT=global
  wires:
  Dead Zone/1 -> MPPT Gain/1
  Switch/1 -> Dead Zone/1  "error"
  Saturation1/1 -> div/2
  Saturation/1 -> div2/2
  Switch1/1 -> Delta_D/1
  on/off/1 -> Switch/2, Switch1/2
  Constant1/1 -> Switch1/3
  Discrete-Time Integrator/1 -> Switch1/1  "Delta_D"
  Constant/1 -> Switch/3
  MPPT Gain/1 -> Discrete-Time Integrator/1
  Add1/1 -> Switch/1  "error"
  div2/1 -> Add1/2, [I_V_MPPT]  "I/V"
  Mean1/1 -> Saturation/1, [Vmean_PV]
  Mean/1 -> div2/1, [Imean_PV]
  div1/1 -> Add1/1, [dI_dV_MPPT]  "dI/dV"
  Trigonometric Function/1 -> div1/2
  div/1 -> div1/1
  deg2rad/1 -> Trigonometric Function/1
  Add/1 -> deg2rad/1
  Fourier1/1 -> Saturation1/1
  Fourier1/2 -> Add/2
  Fourier/2 -> Add/1
  V_PV/1 -> Mean1/1, Fourier1/1
  I_PV/1 -> Mean/1, Fourier/1
  Fourier/1 -> div/1
  [dI_dV_MPPT] -> Mux2/1  "dI/dV"
  Gain/1 -> Mux2/2  "-I/V"
  Mux2/1 -> MPPT Algorithm/1  "dI/dV     -I/V (magenta)"
  [I_V_MPPT] -> Gain/1  "I_V"

== system ACDCMG_woPV/Boost converter DC //CD 2 5 kHz - 300V 1/MPPT Controller using  "Incremental Conductance + Integral Regulator "  technique /MPPT ==
  note: Maximum power point tracking by incremental conductance method
      | --------------------------------------------------------------
      | Maximum power point is obtained when dP/dV=0  where P= V*I
      | -> d(V*I)/dV = I + V*dI/dV = 0
      | -> dI/dV = -I/V
      |
      | dI, dV  = fundamental components of I and V ripples measured with a sliding time window T_MPPT
      | I , V   = mean values of V and I measured with a sliding time window T_MPPT
      |
      | The integral regulator minimizes the error (dI/dV + I/V)
      | Regulator output = Duty cycle correction
  V_PV : Inport
  I_PV : Inport  Port=2
  on/off : Inport  Port=3
  Add : Sum  Inputs=+-
  Add1 : Sum
  Constant : Constant  Value=0
  Constant1 : Constant  Value=0
  Dead Zone : DeadZone  LowerValue=-0.05  UpperValue=0.05  SaturateOnIntegerOverflow=on
  Discrete-Time Integrator : DiscreteIntegrator  SampleTime=Ts_Control  LimitOutput=on  UpperSaturationLimit=1  LowerSaturationLimit=-1  ICPrevOutput=DiscIntNeverNeededParam  ICPrevScaledInput=DiscIntNeverNeededParam
  Fourier : powerlib_meascontrol/Measurements/Fourier  Freq=1/T_MPPT  n=1  InInit=[0, 0]  Ts=Ts_Control
  Fourier1 : powerlib_meascontrol/Measurements/Fourier  Freq=1/T_MPPT  n=1  InInit=[0, 0]  Ts=Ts_Control
  Gain : Gain  Gain=-1
  MPPT Gain : Gain  Gain=5
  MPPT Algorithm : Scope
  Mean : powerlib_meascontrol/Measurements/Mean  Freq=1/T_MPPT  Vinit=0  Ts=Ts_Control
  Mean1 : powerlib_meascontrol/Measurements/Mean  Freq=1/T_MPPT  Vinit=0  Ts=Ts_Control
  Mux2 : Mux  Inputs=2
  Saturation : Saturate  UpperLimit=inf  LowerLimit=eps
  Saturation1 : Saturate  UpperLimit=inf  LowerLimit=eps
  Switch : Switch  Threshold=0.5
  Switch1 : Switch  Threshold=0.5
  Trigonometric Function : Trigonometry  Operator=cos
  deg2rad : Gain  Gain=pi/180
  div : Product  Inputs=*/  RndMeth=Zero
  div1 : Product  Inputs=**  RndMeth=Zero
  div2 : Product  Inputs=*/  RndMeth=Zero
  Delta_D : Outport  VectorParamsAs1DForOutWhenUnconnected=off
  tag scope: I_V_MPPT=global, Imean_PV=global, Vmean_PV=global, dI_dV_MPPT=global
  wires:
  Dead Zone/1 -> MPPT Gain/1
  Switch/1 -> Dead Zone/1  "error"
  Saturation1/1 -> div/2
  Saturation/1 -> div2/2
  Switch1/1 -> Delta_D/1
  on/off/1 -> Switch/2, Switch1/2
  Constant1/1 -> Switch1/3
  Discrete-Time Integrator/1 -> Switch1/1  "Delta_D"
  Constant/1 -> Switch/3
  MPPT Gain/1 -> Discrete-Time Integrator/1
  Add1/1 -> Switch/1  "error"
  div2/1 -> Add1/2, [I_V_MPPT]  "I/V"
  Mean1/1 -> Saturation/1, [Vmean_PV]
  Mean/1 -> div2/1, [Imean_PV]
  div1/1 -> Add1/1, [dI_dV_MPPT]  "dI/dV"
  Trigonometric Function/1 -> div1/2
  div/1 -> div1/1
  deg2rad/1 -> Trigonometric Function/1
  Add/1 -> deg2rad/1
  Fourier1/1 -> Saturation1/1
  Fourier1/2 -> Add/2
  Fourier/2 -> Add/1
  V_PV/1 -> Mean1/1, Fourier1/1
  I_PV/1 -> Mean/1, Fourier/1
  Fourier/1 -> div/1
  [dI_dV_MPPT] -> Mux2/1  "dI/dV"
  Gain/1 -> Mux2/2  "-I/V"
  Mux2/1 -> MPPT Algorithm/1  "dI/dV     -I/V (magenta)"
  [I_V_MPPT] -> Gain/1  "I_V"

== system ACDCMG_woPV/Bus_AC//DC3/Battery system/Ripple Calculations ==
  Signal : Inport
  Reset : Inport  Port=2
  0 : Constant  Value=2
  1 : Constant  Value=2
  Display10 : Display
  Display2 : Display
  Mean1 : powerlib_meascontrol/Measurements/Mean  Freq=10  Vinit=0  Ts=0
  MinMax Running Resettable : simulink/Math Operations/MinMax Running Resettable  Function=max  vinit=0.0
  MinMax Running Resettable1 : simulink/Math Operations/MinMax Running Resettable  Function=min  vinit=0.0
  Product : Product
  Product1 : Product
  Sum : Sum  Inputs=|+-
  Sum1 : Sum  Inputs=|-+
  Switch1 : Switch  Criteria=u2 > Threshold
  Switch2 : Switch  Criteria=u2 > Threshold
  Switch3 : Switch  Criteria=u2 > Threshold
  Ripple in Buck : Outport  VectorParamsAs1DForOutWhenUnconnected=off
  Ripple in Boost : Outport  Port=2  VectorParamsAs1DForOutWhenUnconnected=off
  wires:
  1/1 -> Product1/2
  [I_ref] -> Switch2/2, Switch3/2
  Product1/1 -> Switch3/3
  0/1 -> Product/2
  Switch2/1 -> Ripple in Buck/1
  Switch3/1 -> Ripple in Boost/1
  Product/1 -> Switch2/1
  Signal/1 -> Mean1/1, MinMax Running Resettable1/1, MinMax Running Resettable/1
  Switch1/1 -> Sum1/2, Sum/2
  MinMax Running Resettable/1 -> Sum/1, Display2/1
  MinMax Running Resettable1/1 -> Sum1/1, Display10/1
  Sum/1 -> Product/1
  Reset/1 -> Switch1/2, MinMax Running Resettable1/2, MinMax Running Resettable/2
  Sum1/1 -> Product1/1
  Mean1/1 -> Switch1/3

== system ACDCMG_woPV/Bus_AC//DC3/PV system/Pmean ==
  Product : Product  RndMeth=Zero
  WkW : Gain  Gain=1/1000
  P : Outport  VectorParamsAs1DForOutWhenUnconnected=off
  V : Outport  Port=2  VectorParamsAs1DForOutWhenUnconnected=off
  wires:
  [Vmean_PV] -> Product/1, V/1
  Product/1 -> WkW/1
  [Imean_PV] -> Product/2
  WkW/1 -> P/1  "Pmean_PV (kW)"

== system ACDCMG_woPV/Grid Bi-directional Converter 1.1 300 (DC) // 150 V (AC) P_nom 3kW/Control of Inverter/Discrete PWM Generator1 ==
  note: Pierre Giroux, Gilbert Sybille
      | Power System Laboratory, IREQ
      | Hydro-Quebec
  note: PWM Generator
  Uref : Inport
  BL4 : Logic  Operator=NOT  Inputs=1
  BL5 : Logic  Operator=NOT  Inputs=1
  Constant : Constant  Value=Internal_Phase
  Constant1 : Constant  Value=Internal
  Data Type Conversion : DataTypeConversion  OutDataTypeStr=double  SaturateOnIntegerOverflow=on  RndMeth=Zero
  Data Type Conversion1 : DataTypeConversion  OutDataTypeStr=boolean  SaturateOnIntegerOverflow=on  RndMeth=Zero
  Data Type Conversion2 : DataTypeConversion  OutDataTypeStr=boolean  SaturateOnIntegerOverflow=on  RndMeth=Zero
  Gain : Gain  Gain=2*pi*Freq  SaturateOnIntegerOverflow=on  OutDataTypeStr=Inherit: Same as input  ParamDataTypeStr=Inherit: Same as input
  Gain2 : Gain  Gain=pi/180  SaturateOnIntegerOverflow=on  OutDataTypeStr=Inherit: Same as input  ParamDataTypeStr=Inherit: Same as input
  Gain3 : Gain  Gain=-1  SaturateOnIntegerOverflow=on  OutDataTypeStr=Inherit: Same as input  ParamDataTypeStr=Inherit: Same as input
  Mux : Mux  Inputs=2
  Mux1 : Mux  Inputs=2
  Mux2 : Mux  Inputs=2
  Product : Product  InputSameDT=on  SaturateOnIntegerOverflow=on  OutDataTypeStr=Inherit: Same as first input
  Relational Operator : RelationalOperator  RndMeth=Nearest  InputSameDT=on
  Relational Operator1 : RelationalOperator  RndMeth=Nearest  InputSameDT=on
  Select1A : Selector  InputPortWidth=Select1_PortWidth  IndexOptions=Index vector (dialog)  Indices=Select1_Elements  OutputSizes=1
  Select1B : Selector  InputPortWidth=Select1_PortWidth  IndexOptions=Index vector (dialog)  Indices=Select1_Elements  OutputSizes=1
  Select3 : Selector  InputPortWidth=Select3_PortWidth  IndexOptions=Index vector (dialog)  Indices=Select3_Elements  OutputSizes=1
  Sum : Sum  Inputs=+++  InputSameDT=on  SaturateOnIntegerOverflow=on  OutDataTypeStr=Inherit: Same as first input
  Switch : Switch  Criteria=u2 > Threshold
  Triangle : simulink/Sources/Repeating Sequence  rep_seq_t=[0 1/Fc/4 3/Fc/4 1/Fc]  rep_seq_y=[0 -1 1 0]
  Trigonometric Function : Trigonometry
  m3 : Constant  Value=Phase
  m4 : Constant  Value=mIndex
  t : DigitalClock  SampleTime=Ts
  Pulses : Outport  VectorParamsAs1DForOutWhenUnconnected=off
  wires:
  Mux2/1 -> Select3/1
  Select1B/1 -> Mux2/2
  Select1A/1 -> Mux2/1
  Mux1/1 -> Select1B/1
  Mux/1 -> Select1A/1
  BL5/1 -> Mux1/2
  BL4/1 -> Mux/2
  Gain3/1 -> Relational Operator1/1
  Triangle/1 -> Relational Operator1/2, Relational Operator/2
  Product/1 -> Switch/1
  Constant1/1 -> Switch/2
  Trigonometric Function/1 -> Product/2
  Sum/1 -> Trigonometric Function/1
  m4/1 -> Product/1
  Constant/1 -> Sum/3
  m3/1 -> Gain2/1
  Gain2/1 -> Sum/2
  Gain/1 -> Sum/1
  t/1 -> Gain/1
  Select3/1 -> Data Type Conversion/1
  Data Type Conversion/1 -> Pulses/1
  Relational Operator/1 -> Data Type Conversion1/1
  Data Type Conversion1/1 -> BL4/1, Mux/1
  Relational Operator1/1 -> Data Type Conversion2/1
  Data Type Conversion2/1 -> BL5/1, Mux1/1
  Switch/1 -> Relational Operator/1, Gain3/1
  Uref/1 -> Switch/3

== system ACDCMG_woPV/Grid Bi-directional Converter 1.1 300 (DC) // 150 V (AC) P_nom 3kW/Control of Inverter/MI Controller ==
  Vabc : Inport
  Demux : Demux  Commented=on  Outputs=3
  Demux1 : Demux  Outputs=3
  Mux : Mux  Inputs=3
  Mux1 : Mux  Inputs=3
  Mux2 : Mux  Inputs=3
  OP max / min : Subsystem
  Product : Product  RndMeth=Zero
  Product1 : Product  RndMeth=Zero
  Product2 : Product  RndMeth=Zero
  Subsystem : Subsystem
  Subsystem1 : Subsystem
  Terminator : Terminator
  Terminator1 : Terminator  Commented=on
  Terminator2 : Terminator  Commented=on
  Terminator3 : Terminator
  Terminator4 : Terminator  Commented=on
  Vab1 : powerlib_extras/Discrete Measurements/Discrete  RMS value  Commented=on  Freq=60  Mag_Init=0  Ts=20e-6
      settings: SourceProductBaseCode=PS
  Vab5 : powerlib_extras/Discrete Measurements/Discrete  RMS value  Commented=on  Freq=60  Mag_Init=0  Ts=20e-6
      settings: SourceProductBaseCode=PS
  Vab6 : powerlib_extras/Discrete Measurements/Discrete  RMS value  Commented=on  Freq=60  Mag_Init=0  Ts=20e-6
      settings: SourceProductBaseCode=PS
  Vabc_inv : Outport  VectorParamsAs1DForOutWhenUnconnected=off
  u / m : Outport  Port=2  VectorParamsAs1DForOutWhenUnconnected=off
  wires:
  Product/1 -> Mux2/1
  Product1/1 -> Mux2/2
  Product2/1 -> Mux2/3
  Mux1/1 -> u / m/1
  Vabc/1 -> Demux/1
  Demux/1 -> Vab6/1
  Demux/2 -> Vab5/1
  Demux/3 -> Vab1/1
  Demux1/1 -> Product/1, Mux1/1
  Demux1/2 -> Product1/1, Mux1/2
  Demux1/3 -> Product2/1, Mux1/3
  Subsystem/1(Va) -> Product/2
  Subsystem/2(Vb) -> Product1/2
  Subsystem/3(Vc) -> Product2/2
  Mux2/1 -> Vabc_inv/1
  Vab6/1 -> Terminator2/1
  Subsystem1/3(wt) -> Terminator/1
  Subsystem1/1(Frec) -> Terminator3/1
  Subsystem1/2(sin_cos) -> Subsystem/1(sin_cos)
  Mux/1 -> Demux1/1
  OP max / min/1(ctrl) -> Mux/3, Mux/1, Mux/2
  Vab5/1 -> Terminator1/1
  Vab1/1 -> Terminator4/1

== system ACDCMG_woPV/Grid Bi-directional Converter 1.1 300 (DC) // 150 V (AC) P_nom 3kW1/Control of Inverter/Discrete PWM Generator1 ==
  note: Pierre Giroux, Gilbert Sybille
      | Power System Laboratory, IREQ
      | Hydro-Quebec
  note: PWM Generator
  Uref : Inport
  BL4 : Logic  Operator=NOT  Inputs=1
  BL5 : Logic  Operator=NOT  Inputs=1
  Constant : Constant  Value=Internal_Phase
  Constant1 : Constant  Value=Internal
  Data Type Conversion : DataTypeConversion  OutDataTypeStr=double  SaturateOnIntegerOverflow=on  RndMeth=Zero
  Data Type Conversion1 : DataTypeConversion  OutDataTypeStr=boolean  SaturateOnIntegerOverflow=on  RndMeth=Zero
  Data Type Conversion2 : DataTypeConversion  OutDataTypeStr=boolean  SaturateOnIntegerOverflow=on  RndMeth=Zero
  Gain : Gain  Gain=2*pi*Freq  SaturateOnIntegerOverflow=on  OutDataTypeStr=Inherit: Same as input  ParamDataTypeStr=Inherit: Same as input
  Gain2 : Gain  Gain=pi/180  SaturateOnIntegerOverflow=on  OutDataTypeStr=Inherit: Same as input  ParamDataTypeStr=Inherit: Same as input
  Gain3 : Gain  Gain=-1  SaturateOnIntegerOverflow=on  OutDataTypeStr=Inherit: Same as input  ParamDataTypeStr=Inherit: Same as input
  Mux : Mux  Inputs=2
  Mux1 : Mux  Inputs=2
  Mux2 : Mux  Inputs=2
  Product : Product  InputSameDT=on  SaturateOnIntegerOverflow=on  OutDataTypeStr=Inherit: Same as first input
  Relational Operator : RelationalOperator  RndMeth=Nearest  InputSameDT=on
  Relational Operator1 : RelationalOperator  RndMeth=Nearest  InputSameDT=on
  Select1A : Selector  InputPortWidth=Select1_PortWidth  IndexOptions=Index vector (dialog)  Indices=Select1_Elements  OutputSizes=1
  Select1B : Selector  InputPortWidth=Select1_PortWidth  IndexOptions=Index vector (dialog)  Indices=Select1_Elements  OutputSizes=1
  Select3 : Selector  InputPortWidth=Select3_PortWidth  IndexOptions=Index vector (dialog)  Indices=Select3_Elements  OutputSizes=1
  Sum : Sum  Inputs=+++  InputSameDT=on  SaturateOnIntegerOverflow=on  OutDataTypeStr=Inherit: Same as first input
  Switch : Switch  Criteria=u2 > Threshold
  Triangle : simulink/Sources/Repeating Sequence  rep_seq_t=[0 1/Fc/4 3/Fc/4 1/Fc]  rep_seq_y=[0 -1 1 0]
  Trigonometric Function : Trigonometry
  m3 : Constant  Value=Phase
  m4 : Constant  Value=mIndex
  t : DigitalClock  SampleTime=Ts
  Pulses : Outport  VectorParamsAs1DForOutWhenUnconnected=off
  wires:
  Mux2/1 -> Select3/1
  Select1B/1 -> Mux2/2
  Select1A/1 -> Mux2/1
  Mux1/1 -> Select1B/1
  Mux/1 -> Select1A/1
  BL5/1 -> Mux1/2
  BL4/1 -> Mux/2
  Gain3/1 -> Relational Operator1/1
  Triangle/1 -> Relational Operator1/2, Relational Operator/2
  Product/1 -> Switch/1
  Constant1/1 -> Switch/2
  Trigonometric Function/1 -> Product/2
  Sum/1 -> Trigonometric Function/1
  m4/1 -> Product/1
  Constant/1 -> Sum/3
  m3/1 -> Gain2/1
  Gain2/1 -> Sum/2
  Gain/1 -> Sum/1
  t/1 -> Gain/1
  Select3/1 -> Data Type Conversion/1
  Data Type Conversion/1 -> Pulses/1
  Relational Operator/1 -> Data Type Conversion1/1
  Data Type Conversion1/1 -> BL4/1, Mux/1
  Relational Operator1/1 -> Data Type Conversion2/1
  Data Type Conversion2/1 -> BL5/1, Mux1/1
  Switch/1 -> Relational Operator/1, Gain3/1
  Uref/1 -> Switch/3
